simulink model "CSAD_PIDcontroller_ny"  (R2016b)
settings: Solver=ode3  StartTime=0.0  StopTime=tend  FixedStep=0.01  RelTol=1e-3  EnableMultiTasking=on
undefined symbols (not defined in the file): C, Cdn, Cdt, Cmn, d, D, depCur, des_pos, E, emfact, eps_c, epsilon, hd, hd2, Hoerner, I_s, k_cc, K_d_psi, K_d_x, K_d_y, K_i_psi, K_i_x, K_i_y, K_omega, K_p_psi, K_p_x, K_p_y, Kp, Kq, Kqr, Kt, Ktr, L, Max_Acceleration, Max_rotation, Max_thrust, moorLineProp, n_c, n_max, p_cc, P_max, Q_f0, Q_max, r0, r_cc, r_dot0, rBottomEnd, Rho, rhoCab, rhoWat, stiffSeafloor, T_psi, T_x, T_y, Thruster, Thruster_control, Thruster_lock, velCur, vessel, vesselABC ... (+7)
libraries: marine_gnc x9, dspmtrx3 x6, simulink x6, simulink_extras x3, marine_hydro x3
(part 5 of 5)

== matlab function CSAD_PIDcontroller_ny/Thrust Allocation  /Thruster control /Thruster 2/Propeller Hydrodynamics/Actual Force and Torque ==
  data: Ta output; n input; Qa output; Kq input; Kt input; Ktr input; Kqr input; Rho input; D input; eps_c input; env input
function [Ta,Qa]= ActualForces(n,Kq,Kt,Ktr,Kqr,Rho,D,eps_c,env)
%#codegen
lambda_c = 0.5+0.5*tanh(eps_c*n/5); % Smooth switching between positive and negative thrust. 5 makes switch happen between -5 and 5
K_TC = Kt*lambda_c+(1-lambda_c)*Ktr;
K_QC = Kq*lambda_c+(1-lambda_c)*Kqr;

Ta = sign(n)*K_TC*Rho*(D^4)*n^2-env;
Qa = sign(n)*K_QC*Rho*(D^5)*n^2-env;

== matlab function CSAD_PIDcontroller_ny/Thrust Allocation  /Thruster control /Thruster 2/Thruster control/Core controller/Core controller: Torque,Power and Combined Torque//Power ==
  data: Qcq output; Qcp output; k_cc input; p_cc input; r_cc input; n input; Qcc output; K_t0 input; K_q0 input; D input; Tr input; rho input; eps_c input; K_t0r input; K_q0r input
function [Qcq,Qcp,Qcc]= CoreControl(k_cc,p_cc,r_cc,n,K_t0,K_q0,D,Tr,rho,eps_c,K_t0r,K_q0r)
%#codegen

lambda_c = 0.5+0.5*tanh(eps_c*n/5);
K_TC = K_t0*lambda_c+(1-lambda_c)*K_t0r;
K_QC = K_q0*lambda_c+(1-lambda_c)*K_q0r;
Qcq = (K_QC/K_TC)*D*Tr;
if n == 0
    Qcp = 0;
else
Qcp = sign(Tr)*K_QC*(abs(Tr)^(3/2))/(sqrt(rho)*D*K_TC^(3/2)*abs(n));
end
alpha_c = exp(-k_cc*abs(p_cc*n)^r_cc);

Qcc = alpha_c*Qcq + (1-alpha_c)*Qcp;

== matlab function CSAD_PIDcontroller_ny/Thrust Allocation  /Thruster control /Thruster 2/Thruster control/MATLAB Function ==
  data: Td input; n_d output; K_t0 input; K_t0r input; rho input; D input; eps_c input; n_c input; n_r input; T_r output
function [n_d,T_r]  = ReferenceGenerator(Td,K_t0,K_t0r,rho,D,eps_c,n_c,n_r)
%#codegen


n_d = sign(Td)*sqrt((abs(Td))/(rho*D^4*K_t0));

lambda_c = 0.5+0.5*tanh(eps_c*n_d/5); % Smooth switching between positive and negative thrust
K_TC = K_t0*lambda_c+(1-lambda_c)*K_t0r;

T_r = sign(n_r)*K_TC*rho*D^4*n_r^2;

== matlab function CSAD_PIDcontroller_ny/Virtual CS Inocean Cat I Drillship 6 DOF/FEM mooring/3 DOF transformation ==
  data: eta input; tau_b output; tau_n input
function tau_b = fcn(eta, tau_n)

% a=[cos(eta(6)),sin(eta(6)),0;
%    -sin(eta(6)),cos(eta(6)),0;
%    0,0,1];    

a = [(cos(eta(6))*cos(eta(5))), (sin(eta(6))*cos(eta(5))), -sin(eta(5));
    (-(sin(eta(6))*cos(eta(4)))+(cos(eta(6))*sin(eta(5))*sin(eta(4)))), ((cos(eta(6))*cos(eta(4)))+(sin(eta(4))*sin(eta(5))*sin(eta(6)))), (cos(eta(5))*sin(eta(4)));
    ((sin(eta(6))*sin(eta(4)))+(cos(eta(6))*cos(eta(4))*sin(eta(5)))), (-(cos(eta(6))*sin(eta(4)))+(sin(eta(5))*sin(eta(6))*cos(eta(4)))), (cos(eta(5))*cos(eta(4)))];

tau = a*tau_n;

% Since it is assumed that the ship has a turret-based mooring system,
% and that all cables are connected to the ceter of the turret
% The origin of the body-fixed reference frame is also placed in this center
% The vector p will be zero, and the crossproduct of tau and p will be
% zero, and tau in roll, pitch and yaw will be zero

tau_b=[tau;0;0;0];

== matlab function CSAD_PIDcontroller_ny/Referance/MATLAB Function ==
  data: omega input; y output; zeta input
function y = fcn(omega,zeta)

y = 2*zeta*omega;

== matlab function CSAD_PIDcontroller_ny/Referance/MATLAB Function1 ==
  data: omega input; y output; zeta input
function y = fcn(omega,zeta)

y = 2*zeta*omega;

== matlab function CSAD_PIDcontroller_ny/Referance/MATLAB Function2 ==
  data: omega input; y output
function y = fcn(omega)

y = omega*omega;

== matlab function CSAD_PIDcontroller_ny/Virtual CS Inocean Cat I Drillship 6 DOF/FEM mooring/scaling_eta ==
  data: u input; y output
function y = fcn(u)

lambda = 90;

y = [u(1)*lambda u(2)*lambda u(3)*lambda]';
end

== matlab function CSAD_PIDcontroller_ny/Virtual CS Inocean Cat I Drillship 6 DOF/FEM mooring/scaling_eta1 ==
  data: u input; y output
function y = fcn(u)

lambda = 90;

y = [u(1)*lambda u(2)*lambda u(3)*lambda u(4) u(5) u(6)]';
end

== matlab function CSAD_PIDcontroller_ny/Virtual CS Inocean Cat I Drillship 6 DOF/FEM mooring/scaling_tau ==
  data: u input; y output
function y = fcn(u)

lambda = 90;
roh_f = 1025;
roh_m = 1000;
roh = roh_f/roh_m;
%(1/roh)*

y = (1/roh)*[u(1)/lambda^3 u(2)/lambda^3 u(3)/lambda^3 u(4)/lambda^4 u(5)/lambda^4 u(6)/lambda^4]';
end

== matlab function CSAD_PIDcontroller_ny/Thrust Allocation  /Thruster control /Thruster 2/Thruster control/Supervisor ==
  data: control input; input input; n input; u output
function u = fcn(control,input,n)
u = 1;
if control == 1
if input == 1
    u = 1;
elseif input == 2
    u = 2;
elseif input == 3 && n > 0.01 || input == 3 && n < -0.01
    u = 3;
elseif input == 4 || input == 3 && n < 0.01 || input == 3 && n > -0.01
    u = 4;
else 
    u = 5;
end
end

if control == 2
if input == 1
    u = 1;
elseif input == 2
    u = 2;
elseif input == 3 && n > 0.01 || input == 3 && n < -0.01
    u = 3;
elseif input == 4 || input == 3 && n < 0.01 || input == 3 && n > -0.01
    u = 4;
else 
    u = 5;
end
end

if control == 3
if input == 1
    u = 1;
elseif input == 2
    u = 2;
elseif input == 3 && n > 0.01 || input == 3 && n < -0.01
    u = 3;
elseif input == 4 || input == 3 && n < 0.01 || input == 3 && n > -0.01
    u = 4;
else 
    u = 5;
end
end

if control == 4
if input == 1
    u = 1;
elseif input == 2
    u = 2;
elseif input == 3 && n > 0.01 || input == 3 && n < -0.01
    u = 3;
elseif input == 4 || input == 3 && n < 0.01 || input == 3 && n > -0.01
    u = 4;
else 
    u = 5;
end
end

if control == 5
if input == 1
    u = 1;
elseif input == 2
    u = 2;
elseif input == 3 && n > 0.01 || input == 3 && n < -0.01
    u = 3;
elseif input == 4 || input == 3 && n < 0.01 || input == 3 && n > -0.01
    u = 4;
else 
    u = 5;
end
end

== matlab function CSAD_PIDcontroller_ny/Thrust Allocation  /Thruster control /Thruster 2/Thruster control/Torque limit ==
  data: Q_max input; Q_c output; P_max input; Q_c0 input; n input
function Q_c = Torquelimit(Q_max, P_max, Q_c0, n)
%#codegen
Q_cm = [abs(Q_c0) Q_max P_max/abs(2*pi*n)];

Q_c = sign(Q_c0)*min(Q_cm);

== matlab function CSAD_PIDcontroller_ny/Thrust Allocation  /Thruster control /Thruster 3/Propeller Hydrodynamics/Actual Force and Torque ==
  data: Ta output; n input; Qa output; Kq input; Kt input; Ktr input; Kqr input; Rho input; D input; eps_c input; env input
function [Ta,Qa]= ActualForces(n,Kq,Kt,Ktr,Kqr,Rho,D,eps_c,env)
%#codegen
lambda_c = 0.5+0.5*tanh(eps_c*n/5); % Smooth switching between positive and negative thrust. 5 makes switch happen between -5 and 5
K_TC = Kt*lambda_c+(1-lambda_c)*Ktr;
K_QC = Kq*lambda_c+(1-lambda_c)*Kqr;

Ta = sign(n)*K_TC*Rho*(D^4)*n^2-env;
Qa = sign(n)*K_QC*Rho*(D^5)*n^2-env;

== matlab function CSAD_PIDcontroller_ny/Thrust Allocation  /Thruster control /Thruster 3/Thruster control/Core controller/Core controller: Torque,Power and Combined Torque//Power ==
  data: Qcq output; Qcp output; k_cc input; p_cc input; r_cc input; n input; Qcc output; K_t0 input; K_q0 input; D input; Tr input; rho input; eps_c input; K_t0r input; K_q0r input
function [Qcq,Qcp,Qcc]= CoreControl(k_cc,p_cc,r_cc,n,K_t0,K_q0,D,Tr,rho,eps_c,K_t0r,K_q0r)
%#codegen

lambda_c = 0.5+0.5*tanh(eps_c*n/5);
K_TC = K_t0*lambda_c+(1-lambda_c)*K_t0r;
K_QC = K_q0*lambda_c+(1-lambda_c)*K_q0r;
Qcq = (K_QC/K_TC)*D*Tr;
if n == 0
    Qcp = 0;
else
Qcp = sign(Tr)*K_QC*(abs(Tr)^(3/2))/(sqrt(rho)*D*K_TC^(3/2)*abs(n));
end
alpha_c = exp(-k_cc*abs(p_cc*n)^r_cc);

Qcc = alpha_c*Qcq + (1-alpha_c)*Qcp;

== matlab function CSAD_PIDcontroller_ny/Thrust Allocation  /Thruster control /Thruster 3/Thruster control/MATLAB Function ==
  data: Td input; n_d output; K_t0 input; K_t0r input; rho input; D input; eps_c input; n_c input; n_r input; T_r output
function [n_d,T_r]  = ReferenceGenerator(Td,K_t0,K_t0r,rho,D,eps_c,n_c,n_r)
%#codegen


n_d = sign(Td)*sqrt((abs(Td))/(rho*D^4*K_t0));

lambda_c = 0.5+0.5*tanh(eps_c*n_d/5); % Smooth switching between positive and negative thrust
K_TC = K_t0*lambda_c+(1-lambda_c)*K_t0r;

T_r = sign(n_r)*K_TC*rho*D^4*n_r^2;

== matlab function CSAD_PIDcontroller_ny/Thrust Allocation  /Thruster control /Thruster 3/Thruster control/Supervisor ==
  data: control input; input input; n input; u output
function u = fcn(control,input,n)
u = 1;
if control == 1
if input == 1
    u = 1;
elseif input == 2
    u = 2;
elseif input == 3 && n > 0.01 || input == 3 && n < -0.01
    u = 3;
elseif input == 4 || input == 3 && n < 0.01 || input == 3 && n > -0.01
    u = 4;
else 
    u = 5;
end
end

if control == 2
if input == 1
    u = 1;
elseif input == 2
    u = 2;
elseif input == 3 && n > 0.01 || input == 3 && n < -0.01
    u = 3;
elseif input == 4 || input == 3 && n < 0.01 || input == 3 && n > -0.01
    u = 4;
else 
    u = 5;
end
end

if control == 3
if input == 1
    u = 1;
elseif input == 2
    u = 2;
elseif input == 3 && n > 0.01 || input == 3 && n < -0.01
    u = 3;
elseif input == 4 || input == 3 && n < 0.01 || input == 3 && n > -0.01
    u = 4;
else 
    u = 5;
end
end

if control == 4
if input == 1
    u = 1;
elseif input == 2
    u = 2;
elseif input == 3 && n > 0.01 || input == 3 && n < -0.01
    u = 3;
elseif input == 4 || input == 3 && n < 0.01 || input == 3 && n > -0.01
    u = 4;
else 
    u = 5;
end
end

if control == 5
if input == 1
    u = 1;
elseif input == 2
    u = 2;
elseif input == 3 && n > 0.01 || input == 3 && n < -0.01
    u = 3;
elseif input == 4 || input == 3 && n < 0.01 || input == 3 && n > -0.01
    u = 4;
else 
    u = 5;
end
end

== matlab function CSAD_PIDcontroller_ny/Thrust Allocation  /Thruster control /Thruster 3/Thruster control/Torque limit ==
  data: Q_max input; Q_c output; P_max input; Q_c0 input; n input
function Q_c = Torquelimit(Q_max, P_max, Q_c0, n)
%#codegen
Q_cm = [abs(Q_c0) Q_max P_max/abs(2*pi*n)];

Q_c = sign(Q_c0)*min(Q_cm);

== matlab function CSAD_PIDcontroller_ny/Thrust Allocation  /Thruster control /Thruster 4/Propeller Hydrodynamics/Actual Force and Torque ==
  data: Ta output; n input; Qa output; Kq input; Kt input; Ktr input; Kqr input; Rho input; D input; eps_c input; env input
function [Ta,Qa]= ActualForces(n,Kq,Kt,Ktr,Kqr,Rho,D,eps_c,env)
%#codegen
lambda_c = 0.5+0.5*tanh(eps_c*n/5); % Smooth switching between positive and negative thrust. 5 makes switch happen between -5 and 5
K_TC = Kt*lambda_c+(1-lambda_c)*Ktr;
K_QC = Kq*lambda_c+(1-lambda_c)*Kqr;

Ta = sign(n)*K_TC*Rho*(D^4)*n^2-env;
Qa = sign(n)*K_QC*Rho*(D^5)*n^2-env;

== matlab function CSAD_PIDcontroller_ny/Thrust Allocation  /Thruster control /Thruster 4/Thruster control/Core controller/Core controller: Torque,Power and Combined Torque//Power ==
  data: Qcq output; Qcp output; k_cc input; p_cc input; r_cc input; n input; Qcc output; K_t0 input; K_q0 input; D input; Tr input; rho input; eps_c input; K_t0r input; K_q0r input
function [Qcq,Qcp,Qcc]= CoreControl(k_cc,p_cc,r_cc,n,K_t0,K_q0,D,Tr,rho,eps_c,K_t0r,K_q0r)
%#codegen

lambda_c = 0.5+0.5*tanh(eps_c*n/5);
K_TC = K_t0*lambda_c+(1-lambda_c)*K_t0r;
K_QC = K_q0*lambda_c+(1-lambda_c)*K_q0r;
Qcq = (K_QC/K_TC)*D*Tr;
if n == 0
    Qcp = 0;
else
Qcp = sign(Tr)*K_QC*(abs(Tr)^(3/2))/(sqrt(rho)*D*K_TC^(3/2)*abs(n));
end
alpha_c = exp(-k_cc*abs(p_cc*n)^r_cc);

Qcc = alpha_c*Qcq + (1-alpha_c)*Qcp;

== matlab function CSAD_PIDcontroller_ny/Thrust Allocation  /Thruster control /Thruster 4/Thruster control/MATLAB Function ==
  data: Td input; n_d output; K_t0 input; K_t0r input; rho input; D input; eps_c input; n_c input; n_r input; T_r output
function [n_d,T_r]  = ReferenceGenerator(Td,K_t0,K_t0r,rho,D,eps_c,n_c,n_r)
%#codegen


n_d = sign(Td)*sqrt((abs(Td))/(rho*D^4*K_t0));

lambda_c = 0.5+0.5*tanh(eps_c*n_d/5); % Smooth switching between positive and negative thrust
K_TC = K_t0*lambda_c+(1-lambda_c)*K_t0r;

T_r = sign(n_r)*K_TC*rho*D^4*n_r^2;

== matlab function CSAD_PIDcontroller_ny/Thrust Allocation  /Thruster control /Thruster 4/Thruster control/Supervisor ==
  data: control input; input input; n input; u output
function u = fcn(control,input,n)
u = 1;
if control == 1
if input == 1
    u = 1;
elseif input == 2
    u = 2;
elseif input == 3 && n > 0.01 || input == 3 && n < -0.01
    u = 3;
elseif input == 4 || input == 3 && n < 0.01 || input == 3 && n > -0.01
    u = 4;
else 
    u = 5;
end
end

if control == 2
if input == 1
    u = 1;
elseif input == 2
    u = 2;
elseif input == 3 && n > 0.01 || input == 3 && n < -0.01
    u = 3;
elseif input == 4 || input == 3 && n < 0.01 || input == 3 && n > -0.01
    u = 4;
else 
    u = 5;
end
end

if control == 3
if input == 1
    u = 1;
elseif input == 2
    u = 2;
elseif input == 3 && n > 0.01 || input == 3 && n < -0.01
    u = 3;
elseif input == 4 || input == 3 && n < 0.01 || input == 3 && n > -0.01
    u = 4;
else 
    u = 5;
end
end

if control == 4
if input == 1
    u = 1;
elseif input == 2
    u = 2;
elseif input == 3 && n > 0.01 || input == 3 && n < -0.01
    u = 3;
elseif input == 4 || input == 3 && n < 0.01 || input == 3 && n > -0.01
    u = 4;
else 
    u = 5;
end
end

if control == 5
if input == 1
    u = 1;
elseif input == 2
    u = 2;
elseif input == 3 && n > 0.01 || input == 3 && n < -0.01
    u = 3;
elseif input == 4 || input == 3 && n < 0.01 || input == 3 && n > -0.01
    u = 4;
else 
    u = 5;
end
end

== matlab function CSAD_PIDcontroller_ny/Thrust Allocation  /Thruster control /Thruster 4/Thruster control/Torque limit ==
  data: Q_max input; Q_c output; P_max input; Q_c0 input; n input
function Q_c = Torquelimit(Q_max, P_max, Q_c0, n)
%#codegen
Q_cm = [abs(Q_c0) Q_max P_max/abs(2*pi*n)];

Q_c = sign(Q_c0)*min(Q_cm);

== matlab function CSAD_PIDcontroller_ny/Thrust Allocation  /Thruster control /Thruster 5/Propeller Hydrodynamics/Actual Force and Torque ==
  data: Ta output; n input; Qa output; Kq input; Kt input; Ktr input; Kqr input; Rho input; D input; eps_c input; env input
function [Ta,Qa]= ActualForces(n,Kq,Kt,Ktr,Kqr,Rho,D,eps_c,env)
%#codegen
lambda_c = 0.5+0.5*tanh(eps_c*n/5); % Smooth switching between positive and negative thrust. 5 makes switch happen between -5 and 5
K_TC = Kt*lambda_c+(1-lambda_c)*Ktr;
K_QC = Kq*lambda_c+(1-lambda_c)*Kqr;

Ta = sign(n)*K_TC*Rho*(D^4)*n^2-env;
Qa = sign(n)*K_QC*Rho*(D^5)*n^2-env;

== matlab function CSAD_PIDcontroller_ny/Thrust Allocation  /Thruster control /Thruster 5/Thruster control/Core controller/Core controller: Torque,Power and Combined Torque//Power ==
  data: Qcq output; Qcp output; k_cc input; p_cc input; r_cc input; n input; Qcc output; K_t0 input; K_q0 input; D input; Tr input; rho input; eps_c input; K_t0r input; K_q0r input
function [Qcq,Qcp,Qcc]= CoreControl(k_cc,p_cc,r_cc,n,K_t0,K_q0,D,Tr,rho,eps_c,K_t0r,K_q0r)
%#codegen

lambda_c = 0.5+0.5*tanh(eps_c*n/5);
K_TC = K_t0*lambda_c+(1-lambda_c)*K_t0r;
K_QC = K_q0*lambda_c+(1-lambda_c)*K_q0r;
Qcq = (K_QC/K_TC)*D*Tr;
if n == 0
    Qcp = 0;
else
Qcp = sign(Tr)*K_QC*(abs(Tr)^(3/2))/(sqrt(rho)*D*K_TC^(3/2)*abs(n));
end
alpha_c = exp(-k_cc*abs(p_cc*n)^r_cc);

Qcc = alpha_c*Qcq + (1-alpha_c)*Qcp;

== matlab function CSAD_PIDcontroller_ny/Thrust Allocation  /Thruster control /Thruster 5/Thruster control/MATLAB Function ==
  data: Td input; n_d output; K_t0 input; K_t0r input; rho input; D input; eps_c input; n_c input; n_r input; T_r output
function [n_d,T_r]  = ReferenceGenerator(Td,K_t0,K_t0r,rho,D,eps_c,n_c,n_r)
%#codegen


n_d = sign(Td)*sqrt((abs(Td))/(rho*D^4*K_t0));

lambda_c = 0.5+0.5*tanh(eps_c*n_d/5); % Smooth switching between positive and negative thrust
K_TC = K_t0*lambda_c+(1-lambda_c)*K_t0r;

T_r = sign(n_r)*K_TC*rho*D^4*n_r^2;

== matlab function CSAD_PIDcontroller_ny/Thrust Allocation  /Thruster control /Thruster 5/Thruster control/Supervisor ==
  data: control input; input input; n input; u output
function u = fcn(control,input,n)
u = 1;
if control == 1
if input == 1
    u = 1;
elseif input == 2
    u = 2;
elseif input == 3 && n > 0.01 || input == 3 && n < -0.01
    u = 3;
elseif input == 4 || input == 3 && n < 0.01 || input == 3 && n > -0.01
    u = 4;
else 
    u = 5;
end
end

if control == 2
if input == 1
    u = 1;
elseif input == 2
    u = 2;
elseif input == 3 && n > 0.01 || input == 3 && n < -0.01
    u = 3;
elseif input == 4 || input == 3 && n < 0.01 || input == 3 && n > -0.01
    u = 4;
else 
    u = 5;
end
end

if control == 3
if input == 1
    u = 1;
elseif input == 2
    u = 2;
elseif input == 3 && n > 0.01 || input == 3 && n < -0.01
    u = 3;
elseif input == 4 || input == 3 && n < 0.01 || input == 3 && n > -0.01
    u = 4;
else 
    u = 5;
end
end

if control == 4
if input == 1
    u = 1;
elseif input == 2
    u = 2;
elseif input == 3 && n > 0.01 || input == 3 && n < -0.01
    u = 3;
elseif input == 4 || input == 3 && n < 0.01 || input == 3 && n > -0.01
    u = 4;
else 
    u = 5;
end
end

if control == 5
if input == 1
    u = 1;
elseif input == 2
    u = 2;
elseif input == 3 && n > 0.01 || input == 3 && n < -0.01
    u = 3;
elseif input == 4 || input == 3 && n < 0.01 || input == 3 && n > -0.01
    u = 4;
else 
    u = 5;
end
end

== matlab function CSAD_PIDcontroller_ny/Thrust Allocation  /Thruster control /Thruster 5/Thruster control/Torque limit ==
  data: Q_max input; Q_c output; P_max input; Q_c0 input; n input
function Q_c = Torquelimit(Q_max, P_max, Q_c0, n)
%#codegen
Q_cm = [abs(Q_c0) Q_max P_max/abs(2*pi*n)];

Q_c = sign(Q_c0)*min(Q_cm);

== matlab function CSAD_PIDcontroller_ny/Thrust Allocation  /Thruster control /Thruster 6/Propeller Hydrodynamics/Actual Force and Torque ==
  data: Ta output; n input; Qa output; Kq input; Kt input; Ktr input; Kqr input; Rho input; D input; eps_c input; env input
function [Ta,Qa]= ActualForces(n,Kq,Kt,Ktr,Kqr,Rho,D,eps_c,env)
%#codegen
lambda_c = 0.5+0.5*tanh(eps_c*n/5); % Smooth switching between positive and negative thrust. 5 makes switch happen between -5 and 5
K_TC = Kt*lambda_c+(1-lambda_c)*Ktr;
K_QC = Kq*lambda_c+(1-lambda_c)*Kqr;

Ta = sign(n)*K_TC*Rho*(D^4)*n^2-env;
Qa = sign(n)*K_QC*Rho*(D^5)*n^2-env;

== matlab function CSAD_PIDcontroller_ny/Thrust Allocation  /Thruster control /Thruster 6/Thruster control/Core controller/Core controller: Torque,Power and Combined Torque//Power ==
  data: Qcq output; Qcp output; k_cc input; p_cc input; r_cc input; n input; Qcc output; K_t0 input; K_q0 input; D input; Tr input; rho input; eps_c input; K_t0r input; K_q0r input
function [Qcq,Qcp,Qcc]= CoreControl(k_cc,p_cc,r_cc,n,K_t0,K_q0,D,Tr,rho,eps_c,K_t0r,K_q0r)
%#codegen

lambda_c = 0.5+0.5*tanh(eps_c*n/5);
K_TC = K_t0*lambda_c+(1-lambda_c)*K_t0r;
K_QC = K_q0*lambda_c+(1-lambda_c)*K_q0r;
Qcq = (K_QC/K_TC)*D*Tr;
if n == 0
    Qcp = 0;
else
Qcp = sign(Tr)*K_QC*(abs(Tr)^(3/2))/(sqrt(rho)*D*K_TC^(3/2)*abs(n));
end
alpha_c = exp(-k_cc*abs(p_cc*n)^r_cc);

Qcc = alpha_c*Qcq + (1-alpha_c)*Qcp;

== matlab function CSAD_PIDcontroller_ny/Thrust Allocation  /Thruster control /Thruster 6/Thruster control/MATLAB Function ==
  data: Td input; n_d output; K_t0 input; K_t0r input; rho input; D input; eps_c input; n_c input; n_r input; T_r output
function [n_d,T_r]  = ReferenceGenerator(Td,K_t0,K_t0r,rho,D,eps_c,n_c,n_r)
%#codegen


n_d = sign(Td)*sqrt((abs(Td))/(rho*D^4*K_t0));

lambda_c = 0.5+0.5*tanh(eps_c*n_d/27); % Smooth switching between positive and negative thrust
K_TC = K_t0*lambda_c+(1-lambda_c)*K_t0r;

T_r = sign(n_r)*K_TC*rho*D^4*n_r^2;

== matlab function CSAD_PIDcontroller_ny/Thrust Allocation  /Thruster control /Thruster 6/Thruster control/Supervisor ==
  data: control input; input input; n input; u output
function u = fcn(control,input,n)
u = 1;
if control == 1
if input == 1
    u = 1;
elseif input == 2
    u = 2;
elseif input == 3 && n > 0.01 || input == 3 && n < -0.01
    u = 3;
elseif input == 4 || input == 3 && n < 0.01 || input == 3 && n > -0.01
    u = 4;
else 
    u = 5;
end
end

if control == 2
if input == 1
    u = 1;
elseif input == 2
    u = 2;
elseif input == 3 && n > 0.01 || input == 3 && n < -0.01
    u = 3;
elseif input == 4 || input == 3 && n < 0.01 || input == 3 && n > -0.01
    u = 4;
else 
    u = 5;
end
end

if control == 3
if input == 1
    u = 1;
elseif input == 2
    u = 2;
elseif input == 3 && n > 0.01 || input == 3 && n < -0.01
    u = 3;
elseif input == 4 || input == 3 && n < 0.01 || input == 3 && n > -0.01
    u = 4;
else 
    u = 5;
end
end

if control == 4
if input == 1
    u = 1;
elseif input == 2
    u = 2;
elseif input == 3 && n > 0.01 || input == 3 && n < -0.01
    u = 3;
elseif input == 4 || input == 3 && n < 0.01 || input == 3 && n > -0.01
    u = 4;
else 
    u = 5;
end
end

if control == 5
if input == 1
    u = 1;
elseif input == 2
    u = 2;
elseif input == 3 && n > 0.01 || input == 3 && n < -0.01
    u = 3;
elseif input == 4 || input == 3 && n < 0.01 || input == 3 && n > -0.01
    u = 4;
else 
    u = 5;
end
end

== matlab function CSAD_PIDcontroller_ny/Thrust Allocation  /Thruster control /Thruster 6/Thruster control/Torque limit ==
  data: Q_max input; Q_c output; P_max input; Q_c0 input; n input
function Q_c = Torquelimit(Q_max, P_max, Q_c0, n)
%#codegen
Q_cm = [abs(Q_c0) Q_max P_max/abs(2*pi*n)];

Q_c = sign(Q_c0)*min(Q_cm);
